simulink model "stateflow_flowterminal"  (R2015b)
settings: Solver=VariableStepAuto  StartTime=0.0  StopTime=10.0  RelTol=1e-3
settings Model: Creator=amyyang  LastModifiedBy=amyyang

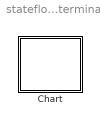
== system stateflow_flowterminal ==
  Chart : Stateflow chart  TreatAsAtomicUnit=on

== stateflow chart stateflow_flowterminal/Chart ==
  note: 不要在多个地方给返回值赋值
  note: 在07b以前的老版本是影响代码生成，会产生多个返回值赋值语句，违反 MISCA-C 1998的规则；
      | 而在08a以后的版本，不会有这个问题。考虑到代码效率，function 右键属性菜单，设置 Function Inline Option为'function'
      | 新版本，但是考虑到流程图的规范，需要遵守这个规则。
  state A = F1(B,C) [function]
    (default) -> (junction 67)
    (junction 67) -> (junction 65) [order 1] : [ B == 0]
    (junction 65) -> (junction 66) [order 1] : [ C == 0]
    (junction 65) -> (junction 63) [order 2] : {
        |  A = 1;
        | }
    (junction 67) -> (junction 72) [order 2] : {
        |  A = 1;
        | }
    (junction 66) -> (junction 75) : {
        |  A = 1;
        | }
  state A = F(B,C) [function]
    (default) -> (junction 40)
    (junction 40) -> (junction 42) [order 1] : [ B == 0]
    (junction 42) -> (junction 44) [order 1] : [ C == 0]
    (junction 42) -> (junction 48) [order 2] : {
        |  D = 1;
        | }
    (junction 40) -> (junction 46) [order 2] : {
        |  D = 1;
        | }
    (junction 44) -> (junction 50) : {
        |  D = 1;
        | }
    (junction 48) -> (junction 46)
    (junction 50) -> (junction 48)
    (junction 46) -> (junction 52) : {
        |  A = D;
        | }
  data: B function_input double; C function_input double; A function_output double; B function_input double; C function_input double; A function_output double
